simulink model "linear_observer_control"  (R2023a)
settings: Solver=VariableStepAuto  StartTime=0.0  StopTime=20  RelTol=1e-3
settings Model: Creator=belov  LastModifiedBy=belov

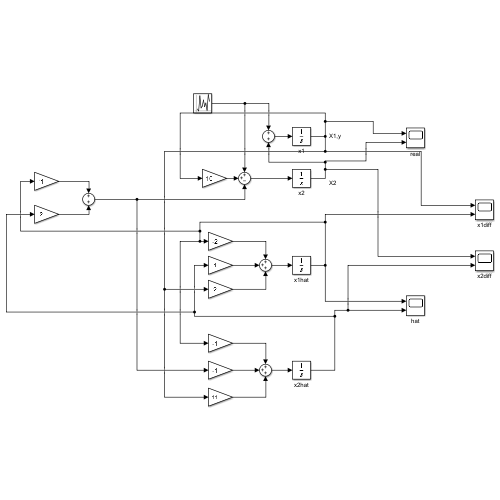
[thumbnail: Simulink's stored preview of the top-level diagram]
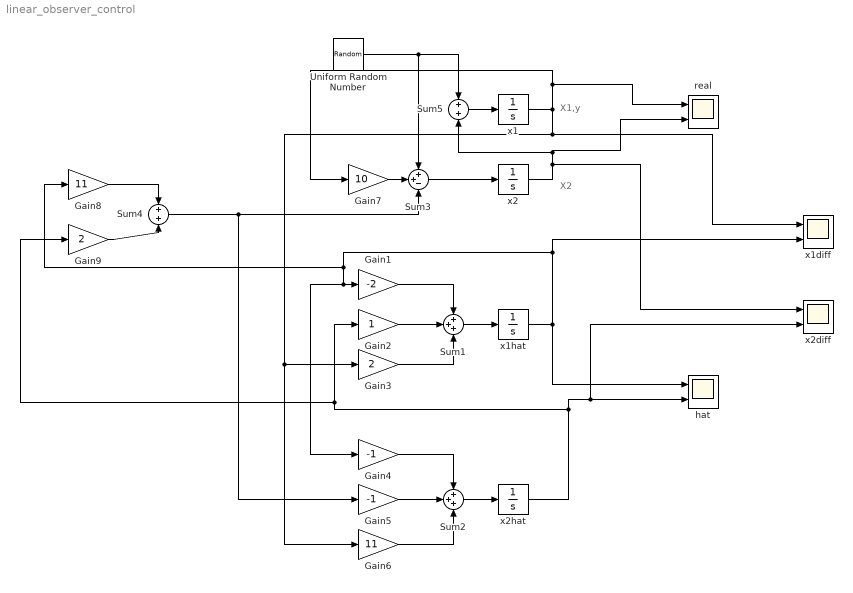
== system linear_observer_control ==
  note: X1,y
  note: X2
  Gain1 : Gain  Gain=-2
  Gain2 : Gain
  Gain3 : Gain  Gain=2
  Gain4 : Gain  Gain=-1
  Gain5 : Gain  Gain=-1
  Gain6 : Gain  Gain=11
  Gain7 : Gain  Gain=10
  Gain8 : Gain  Gain=11
  Gain9 : Gain  Gain=2
  Sum1 : Sum  Inputs=+++
  Sum2 : Sum  Inputs=+++
  Sum3 : Sum  Inputs=++-
  Sum4 : Sum
  Sum5 : Sum
  Uniform Random Number : UniformRandomNumber  Minimum=-0.05  Maximum=0.05  SampleTime=0.1
  hat : Scope  NumInputPorts=2
  real : Scope  NumInputPorts=2
  x1 : Integrator  InitialCondition=1
  x1diff : Scope  NumInputPorts=2
  x1hat : Integrator
  x2 : Integrator
  x2diff : Scope  NumInputPorts=2
  x2hat : Integrator
  wires:
  Gain6/1 -> Sum2/3
  Gain3/1 -> Sum1/3
  x2/1 -> x2diff/1, Sum5/2, real/2
  x1/1 -> real/1, Gain7/1, x1diff/1, Gain6/1, Gain3/1
  Sum4/1 -> Sum3/3, Gain5/1
  Gain7/1 -> Sum3/2
  Sum3/1 -> x2/1
  Sum2/1 -> x2hat/1
  Sum1/1 -> x1hat/1
  Gain1/1 -> Sum1/1
  Gain5/1 -> Sum2/2
  Gain2/1 -> Sum1/2
  x1hat/1 -> x1diff/2, Gain8/1, Gain4/1, Gain1/1, hat/1
  x2hat/1 -> x2diff/2, hat/2, Gain9/1, Gain2/1
  Gain4/1 -> Sum2/1
  Gain9/1 -> Sum4/2
  Gain8/1 -> Sum4/1
  Sum5/1 -> x1/1
  Uniform Random Number/1 -> Sum3/1, Sum5/1
